simulink model "Simulation"  (R2019b)
settings: Solver=VariableStepAuto  StartTime=0.0  StopTime=150  RelTol=1e-3
values from neighbouring files (symbols this model uses):
  A = [1 1 1 1 ... (first row only)    [Parameters.m]
  actuator_calculator = [ ... (first row only)    [Parameters.m]
  cl = 0.0000002    (= 2e-07)    [Parameters.m]
  g = -9.81    [Parameters.m]
  ground_level = 0    [Parameters.m]
  Ixx = 0.2    [Parameters.m]
  Iyy = 0.2    [Parameters.m]
  Izz = 0.2    [Parameters.m]
  m = 2.2    [Parameters.m]
  maxLiftForce = maxRPM^2 * cl    (= 20)    [Parameters.m]
  P = [0 0 0 0 ... (first row only)    [Parameters.m]
  Pos_init = [0;0;0]    [Parameters.m]
  Vel_init = [0;0;0]    [Parameters.m]
libraries: simulink x12, sharedtransform x6, dspsolvers x2, sharedutil x1, aerolibutil x1, aerolibnav x1
settings Model: Creator=Szabolcs  LastModifiedBy=Szabolcs
settings SolverCC: ZeroCrossAlgorithm=Adaptive
settings DebuggingCC: IgnoredZcDiagnostic=none

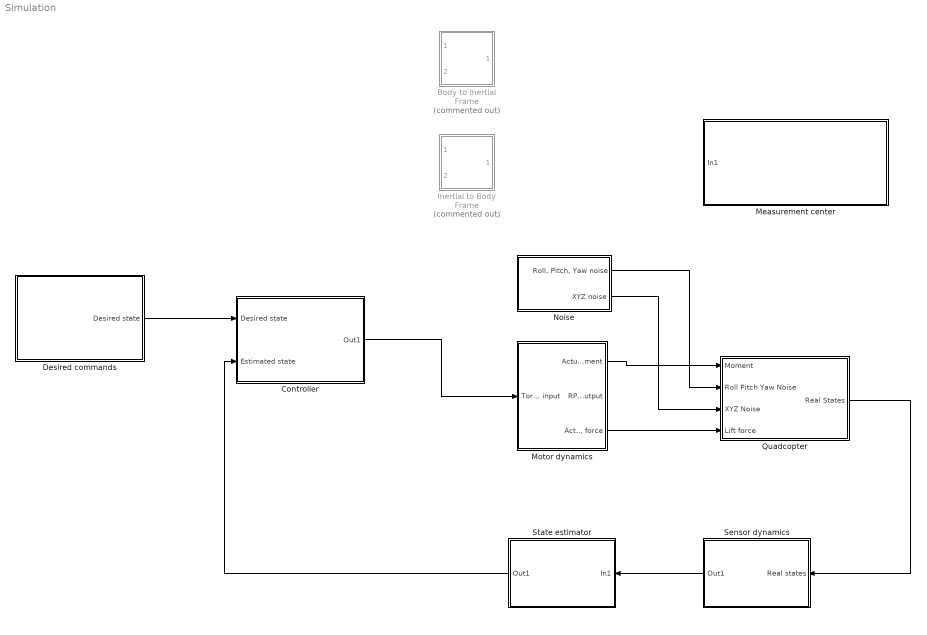
== system Simulation ==
  Body to Inertial Frame : Subsystem  Commented=on
  Controller : Subsystem
  Desired commands : Subsystem
  Inertial to Body Frame : Subsystem  Commented=on
  Measurement center : Subsystem
  Motor dynamics : Subsystem
  Noise : Subsystem
  Quadcopter : Subsystem
  Sensor dynamics : Subsystem
  State estimator : Subsystem
  wires:
  Quadcopter/1(Real States) -> Sensor dynamics/1(Real states)
  Sensor dynamics/1(Out1) -> State estimator/1(In1)
  Motor dynamics/3(Actuator Lift force) -> Quadcopter/4(Lift force)
  Motor dynamics/1(Actuator Moment) -> Quadcopter/1(Moment)
  Noise/2(XYZ noise) -> Quadcopter/3(XYZ Noise)
  Noise/1("Roll, Pitch, Yaw noise") -> Quadcopter/2(Roll Pitch Yaw Noise)
  Desired commands/1(Desired state) -> Controller/1(Desired state)
  State estimator/1(Out1) -> Controller/2(Estimated state)
  Controller/1(Out1) -> Motor dynamics/1(Torque input)

== system Simulation/Body to Inertial Frame ==
  Angles : Inport
  Inertial Vector : Inport  Port=2
  Matrix Multiply : Product  Multiplication=Matrix(*)
  Rotation Angles to Direction Cosine Matrix : sharedtransform/Rotation Angles to Direction Cosine Matrix  rotationOrder=ZYX  aMode=aMode
      settings: SourceProductBaseCode=AE
  Selector3 : Selector  InputPortWidth=3  IndexOptions=Index vector (dialog)  Indices=[3 2 1]  OutputSizes=1
  Transpose : Math  Operator=transpose  RndMeth=Zero  SaturateOnIntegerOverflow=on
  Body Vector : Outport
  wires:
  Rotation Angles to Direction Cosine Matrix/1 -> Transpose/1
  Selector3/1 -> Rotation Angles to Direction Cosine Matrix/1
  Angles/1 -> Selector3/1
  Matrix Multiply/1 -> Body Vector/1
  Inertial Vector/1 -> Matrix Multiply/2
  Transpose/1 -> Matrix Multiply/1

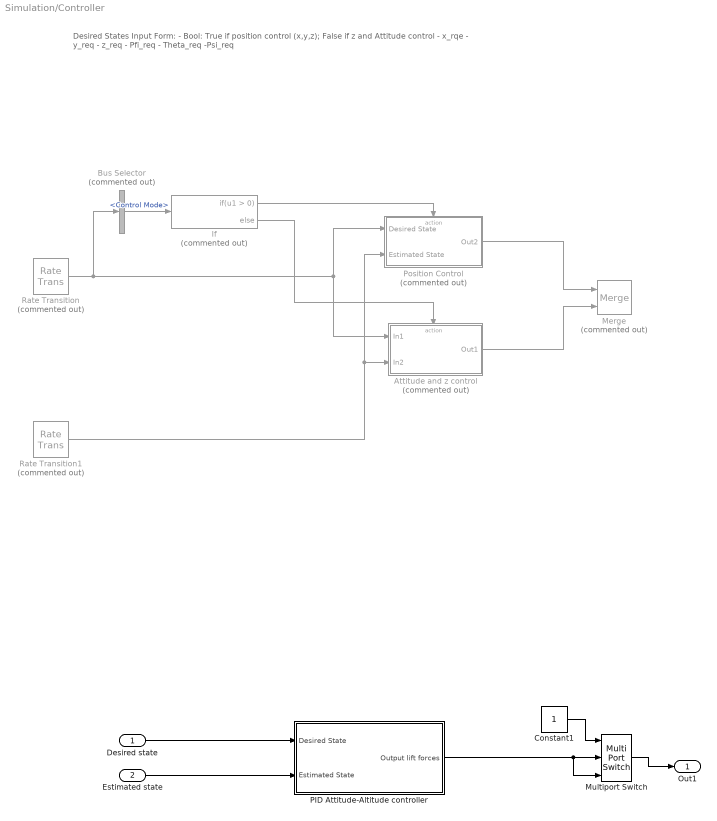
== system Simulation/Controller ==
  note: Desired States Input Form:
      | - Bool: True if position control (x,y,z); False if z and Attitude control
      | - x_rqe
      | - y_req
      | - z_req
      | - Pfi_req
      | - Theta_req
      | -Psi_req
  Desired state : Inport
  Estimated state : Inport  Port=2
  Attitude and z control : Subsystem  Commented=on  TreatAsAtomicUnit=on
  Bus Selector : BusSelector  Commented=on  OutputSignals=Control Mode
  Constant1 : Constant
  If : If  Commented=on
  Merge : Merge  Commented=on
  Multiport Switch : MultiPortSwitch  Inputs=2
  PID Attitude-Altitude controller : Subsystem
  Position Control : Subsystem  Commented=on  TreatAsAtomicUnit=on
  Rate Transition : RateTransition  Commented=on
  Rate Transition1 : RateTransition  Commented=on
  Out1 : Outport
  wires:
  Attitude and z control/1(Out1) -> Merge/2
  Position Control/1(Out2) -> Merge/1
  Bus Selector/1 -> If/1  "<Control Mode>"
  If/1 -> Position Control/Action
  If/2 -> Attitude and z control/Action
  Rate Transition/1 -> Position Control/1(Desired State), Attitude and z control/1(In1), Bus Selector/1
  Rate Transition1/1 -> Position Control/2(Estimated State), Attitude and z control/2(In2)
  Multiport Switch/1 -> Out1/1
  Constant1/1 -> Multiport Switch/1
  Desired state/1 -> PID Attitude-Altitude controller/1(Desired State)
  Estimated state/1 -> PID Attitude-Altitude controller/2(Estimated State)
  PID Attitude-Altitude controller/1(Output lift forces) -> Multiport Switch/3, Multiport Switch/2

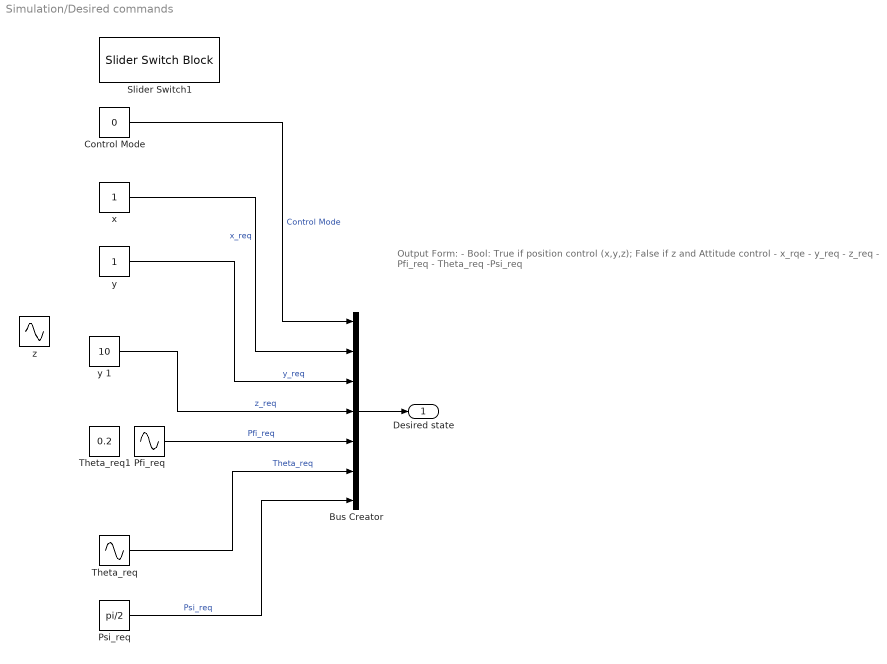
== system Simulation/Desired commands ==
  note: Output Form:
      | - Bool: True if position control (x,y,z); False if z and Attitude control
      | - x_rqe
      | - y_req
      | - z_req
      | - Pfi_req
      | - Theta_req
      | -Psi_req
  Bus Creator : BusCreator  Inputs=7
  Control Mode : Constant  Value=0
  Pfi_req : Sin  Amplitude=pi/6  Frequency=pi/10  SampleTime=0
  Psi_req : Constant  Value=pi/2
  Slider Switch1 : SliderSwitchBlock
      settings: Values={{'Off', 'On'}, [0 1]}
  Theta_req : Sin  Amplitude=pi/6  Frequency=pi/10  SampleTime=0
  Theta_req1 : Constant  Value=0.2
  x : Constant
  "y " : Constant
  y 1 : Constant  Value=10
  z : Sin  Amplitude=2  Bias=4  Frequency=pi/2  SampleTime=0
  Desired state : Outport
  wires:
  Psi_req/1 -> Bus Creator/7  "Psi_req"
  Bus Creator/1 -> Desired state/1
  Theta_req/1 -> Bus Creator/6  "Theta_req"
  "y "/1 -> Bus Creator/3  "y_req"
  Control Mode/1 -> Bus Creator/1  "Control Mode"
  x/1 -> Bus Creator/2  "x_req"
  y 1/1 -> Bus Creator/4  "z_req"
  Pfi_req/1 -> Bus Creator/5  "Pfi_req"

== system Simulation/Inertial to Body Frame ==
  Angles : Inport
  Inertial Vector : Inport  Port=2
  Matrix Multiply : Product  Multiplication=Matrix(*)
  Rotation Angles to Direction Cosine Matrix : sharedtransform/Rotation Angles to Direction Cosine Matrix  rotationOrder=ZYX  aMode=aMode
      settings: SourceProductBaseCode=AE
  Selector3 : Selector  InputPortWidth=3  IndexOptions=Index vector (dialog)  Indices=[3 2 1]  OutputSizes=1
  Body Vector : Outport
  wires:
  Selector3/1 -> Rotation Angles to Direction Cosine Matrix/1
  Angles/1 -> Selector3/1
  Matrix Multiply/1 -> Body Vector/1
  Inertial Vector/1 -> Matrix Multiply/2
  Rotation Angles to Direction Cosine Matrix/1 -> Matrix Multiply/1

== system Simulation/Measurement center ==
  In1 : Inport

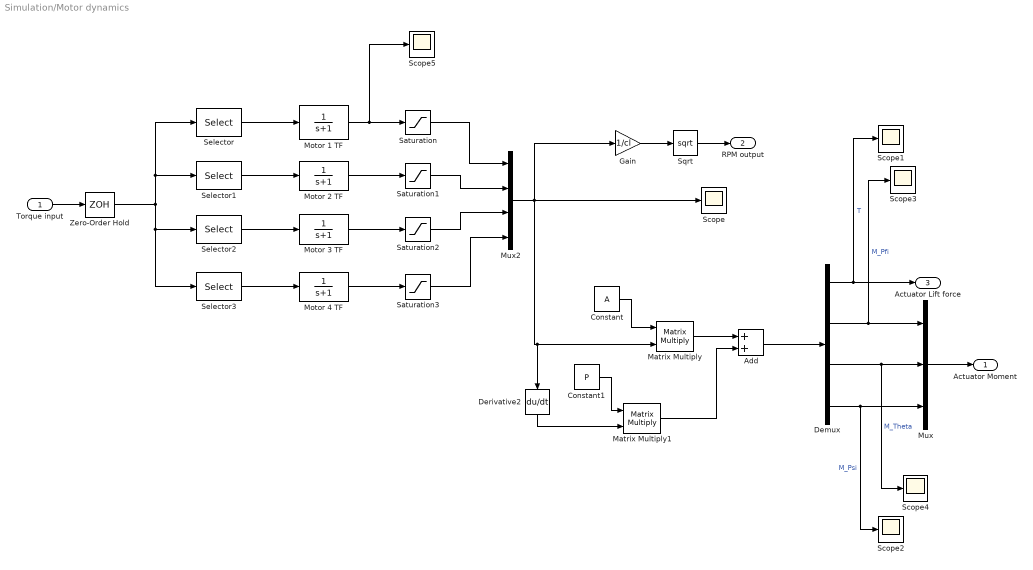
== system Simulation/Motor dynamics ==
  Torque input : Inport
  Add : Sum
  Constant : Constant  Value=A
  Constant1 : Constant  Value=P
  Demux : Demux
  Derivative2 : Derivative
  Gain : Gain  Gain=1/cl
  Matrix Multiply : Product  Multiplication=Matrix(*)
  Matrix Multiply1 : Product  Multiplication=Matrix(*)
  Motor 1 TF : TransferFcn  Denominator=[1 1]
  Motor 2 TF : TransferFcn  Denominator=[1 1]
  Motor 3 TF : TransferFcn  Denominator=[1 1]
  Motor 4 TF : TransferFcn  Denominator=[1 1]
  Mux : Mux  Inputs=3
  Mux2 : Mux
  Saturation{,1..3} (4 alike) : Saturate  UpperLimit=20  LowerLimit=0
  Scope{,1..5} (6 alike) : Scope
  Selector : Selector  InputPortWidth=4  IndexOptions=Index vector (dialog)  Indices=1  OutputSizes=1
  Selector1 : Selector  InputPortWidth=4  IndexOptions=Index vector (dialog)  Indices=2  OutputSizes=1
  Selector2 : Selector  InputPortWidth=4  IndexOptions=Index vector (dialog)  Indices=3  OutputSizes=1
  Selector3 : Selector  InputPortWidth=4  IndexOptions=Index vector (dialog)  Indices=4  OutputSizes=1
  Sqrt : Sqrt  SaturateOnIntegerOverflow=on
  Zero-Order Hold : ZeroOrderHold  SampleTime=0.01
  Actuator Moment : Outport
  RPM output : Outport  Port=2
  Actuator Lift force : Outport  Port=3
  wires:
  Selector/1 -> Motor 1 TF/1
  Selector1/1 -> Motor 2 TF/1
  Zero-Order Hold/1 -> Selector3/1, Selector2/1, Selector1/1, Selector/1
  Torque input/1 -> Zero-Order Hold/1
  Saturation/1 -> Mux2/1
  Saturation1/1 -> Mux2/2
  Selector3/1 -> Motor 4 TF/1
  Saturation3/1 -> Mux2/4
  Saturation2/1 -> Mux2/3
  Motor 1 TF/1 -> Scope5/1, Saturation/1
  Motor 3 TF/1 -> Saturation2/1
  Motor 4 TF/1 -> Saturation3/1
  Motor 2 TF/1 -> Saturation1/1
  Selector2/1 -> Motor 3 TF/1
  Mux2/1 -> Gain/1, Derivative2/1, Matrix Multiply/2, Scope/1
  Constant/1 -> Matrix Multiply/1
  Constant1/1 -> Matrix Multiply1/1
  Derivative2/1 -> Matrix Multiply1/2
  Mux/1 -> Actuator Moment/1
  Sqrt/1 -> RPM output/1
  Gain/1 -> Sqrt/1
  Matrix Multiply1/1 -> Add/2
  Demux/1 -> Scope1/1, Actuator Lift force/1  "T"
  Demux/4 -> Scope2/1, Mux/3  "M_Psi"
  Demux/2 -> Scope3/1, Mux/1  "M_Pfi"
  Demux/3 -> Mux/2, Scope4/1  "M_Theta"
  Matrix Multiply/1 -> Add/1
  Add/1 -> Demux/1

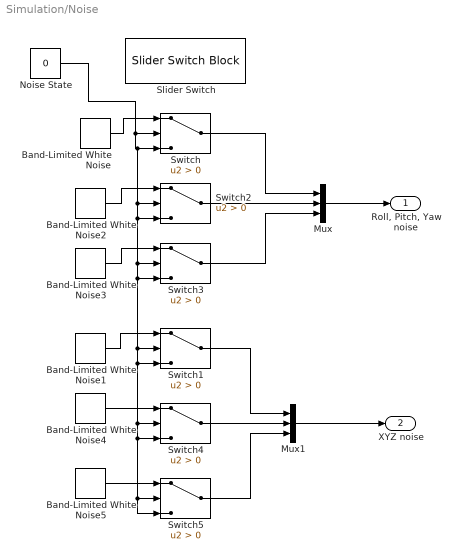
== system Simulation/Noise ==
  Band-Limited White Noise{,1..5} (6 alike) : simulink/Sources/Band-Limited White Noise  Cov=[1]  Ts=0.1  seed=[23341]
  Mux : Mux  Inputs=3
  Mux1 : Mux  Inputs=3
  Noise State : Constant  Value=0
  Slider Switch : SliderSwitchBlock
      settings: Values={{'Off', 'On'}, [0 1]}
  Switch{,1..5} (6 alike) : Switch  Criteria=u2 > Threshold
  "Roll, Pitch, Yaw noise" : Outport
  XYZ noise : Outport  Port=2
  wires:
  Noise State/1 -> Switch2/2, Switch2/3, Switch3/2, Switch3/3, Switch5/3, Switch5/2, Switch4/3, Switch4/2, Switch1/3, Switch1/2, Switch/3, Switch/2
  Band-Limited White Noise/1 -> Switch/1
  Band-Limited White Noise1/1 -> Switch1/1
  Mux/1 -> "Roll, Pitch, Yaw noise"/1
  Switch/1 -> Mux/1
  Switch2/1 -> Mux/2
  Switch3/1 -> Mux/3
  Band-Limited White Noise3/1 -> Switch3/1
  Band-Limited White Noise2/1 -> Switch2/1
  Switch4/1 -> Mux1/2
  Switch1/1 -> Mux1/1
  Switch5/1 -> Mux1/3
  Mux1/1 -> XYZ noise/1
  Band-Limited White Noise4/1 -> Switch4/1
  Band-Limited White Noise5/1 -> Switch5/1

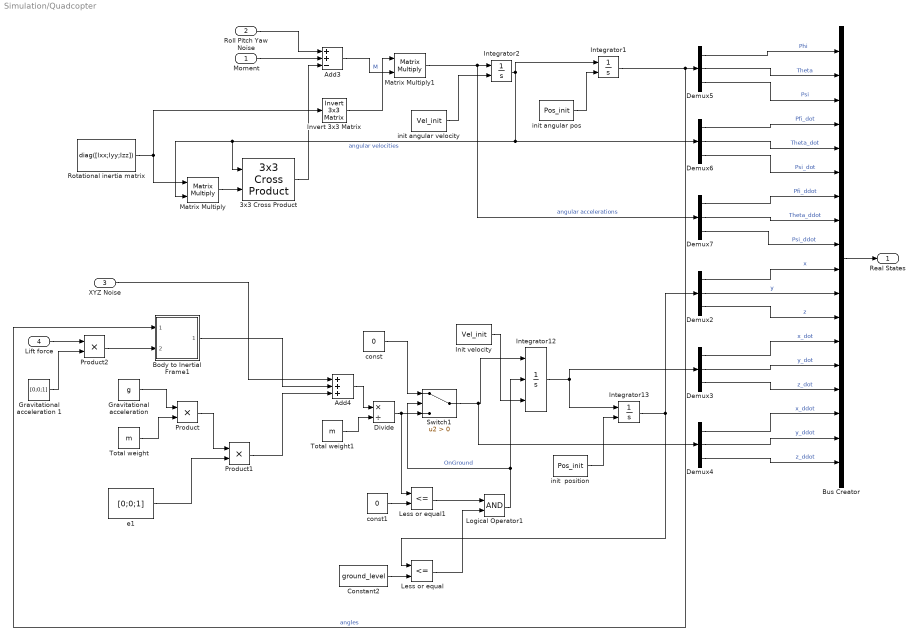
== system Simulation/Quadcopter ==
  Moment : Inport
  Roll Pitch Yaw Noise : Inport  Port=2
  XYZ Noise : Inport  Port=3
  Lift force : Inport  Port=4
  3x3 Cross Product : sharedutil/3x3 Cross Product  aMode=aMode
      settings: SourceProductBaseCode=AE
  Add3 : Sum  Inputs=++-
  Add4 : Sum  Inputs=+++
  Body to Inertial Frame1 : Subsystem
  Bus Creator : BusCreator  Inputs=18
  Constant2 : Constant  Value=ground_level
  Demux{2..7} (6 alike) : Demux  Outputs=3
  Divide : Product  Inputs=*/
  "Gravitational acceleration " : Constant  Value=g
  Gravitational acceleration 1 : Constant  Value=[0;0;1]
  Init velocity : Constant  Value=Vel_init
  Integrator1 : Integrator  InitialConditionSource=external
  Integrator12 : Integrator  ExternalReset=rising  InitialConditionSource=external
  Integrator13 : Integrator  InitialConditionSource=external
  Integrator2 : Integrator  InitialConditionSource=external
  Invert 3x3 Matrix : aerolibutil/Invert  3x3 Matrix
  Less or equal : RelationalOperator  Operator=<=  OutDataTypeStr=boolean  RndMeth=Simplest
  Less or equal1 : RelationalOperator  Operator=<=  OutDataTypeStr=boolean  RndMeth=Simplest
  Logical Operator1 : Logic  AllPortsSameDT=off  OutDataTypeStr=boolean
  Matrix Multiply : Product  Multiplication=Matrix(*)
  Matrix Multiply1 : Product  Multiplication=Matrix(*)
  Product : Product
  Product1 : Product
  Product2 : Product
  Rotational inertia matrix : Constant  Value=diag([Ixx;Iyy;Izz])
  Switch1 : Switch  Criteria=u2 > Threshold
  Total weight : Constant  Value=m
  Total weight1 : Constant  Value=m
  const : Constant  Value=0
  const1 : Constant  Value=0
  e1 : Constant  Value=[0;0;1]
  init  position : Constant  Value=Pos_init
  init angular pos : Constant  Value=Pos_init
  init angular velocity : Constant  Value=Vel_init
  Real States : Outport
  wires:
  Constant2/1 -> Less or equal/2
  Total weight1/1 -> Divide/2
  Integrator13/1 -> Less or equal/1, Demux2/1
  Divide/1 -> Less or equal1/1, Switch1/3
  const1/1 -> Less or equal1/2
  Product1/1 -> Add4/3
  e1/1 -> Product1/2
  Product/1 -> Product1/1
  Switch1/1 -> Demux4/1, Integrator12/1
  Logical Operator1/1 -> Switch1/2, Integrator12/2  "OnGround"
  Total weight/1 -> Product/2
  const/1 -> Switch1/1
  Body to Inertial Frame1/1(Body Vector) -> Add4/2
  Less or equal1/1 -> Logical Operator1/1
  "Gravitational acceleration "/1 -> Product/1
  Less or equal/1 -> Logical Operator1/2
  Add4/1 -> Divide/1
  XYZ Noise/1 -> Add4/1
  Integrator2/1 -> Integrator1/1, Demux6/1, 3x3 Cross Product/1, Matrix Multiply/2  "angular velocities"
  Integrator1/1 -> Body to Inertial Frame1/1(Angles), Demux5/1  "angles"
  Rotational inertia matrix/1 -> Matrix Multiply/1, Invert 3x3 Matrix/1
  Matrix Multiply1/1 -> Integrator2/1, Demux7/1  "angular accelerations"
  Roll Pitch Yaw Noise/1 -> Add3/1
  Moment/1 -> Add3/2
  Add3/1 -> Matrix Multiply1/2  "M"
  Invert 3x3 Matrix/1 -> Matrix Multiply1/1
  3x3 Cross Product/1 -> Add3/3
  Matrix Multiply/1 -> 3x3 Cross Product/2
  init angular velocity/1 -> Integrator2/2
  init angular pos/1 -> Integrator1/2
  Init velocity/1 -> Integrator12/3
  init  position/1 -> Integrator13/2
  Integrator12/1 -> Integrator13/1, Demux3/1
  Bus Creator/1 -> Real States/1
  Demux5/1 -> Bus Creator/1  "Phi"
  Demux5/2 -> Bus Creator/2  "Theta"
  Demux5/3 -> Bus Creator/3  "Psi"
  Demux6/1 -> Bus Creator/4  "Pfi_dot"
  Demux6/2 -> Bus Creator/5  "Theta_dot"
  Demux6/3 -> Bus Creator/6  "Psi_dot"
  Demux7/1 -> Bus Creator/7  "Pfi_ddot"
  Demux7/2 -> Bus Creator/8  "Theta_ddot"
  Demux7/3 -> Bus Creator/9  "Psi_ddot"
  Demux2/1 -> Bus Creator/10  "x"
  Demux2/2 -> Bus Creator/11  "y"
  Demux2/3 -> Bus Creator/12  "z"
  Demux3/1 -> Bus Creator/13  "x_dot"
  Demux3/2 -> Bus Creator/14  "y_dot"
  Demux3/3 -> Bus Creator/15  "z_dot"
  Demux4/1 -> Bus Creator/16  "x_ddot"
  Demux4/2 -> Bus Creator/17  "y_ddot"
  Demux4/3 -> Bus Creator/18  "z_ddot"
  Lift force/1 -> Product2/1
  Product2/1 -> Body to Inertial Frame1/2(Inertial Vector)
  Gravitational acceleration 1/1 -> Product2/2

== system Simulation/Sensor dynamics ==
  Real states : Inport
  Advanced sensor behavious simulation : Constant  Value=0
  Detailed sensor behaviour : Subsystem
  Simplified sensor behaviour : Subsystem
  Slider Switch : SliderSwitchBlock
      settings: Values={{'Off', 'On'}, [0 1]}
  Switch1 : Switch  Criteria=u2 > Threshold
  Out1 : Outport
  wires:
  Switch1/1 -> Out1/1
  Advanced sensor behavious simulation/1 -> Switch1/2
  Real states/1 -> Simplified sensor behaviour/1(Real states), Detailed sensor behaviour/1(In1)
  Simplified sensor behaviour/1(Sensor output) -> Switch1/1, Switch1/3

== system Simulation/State estimator ==
  In1 : Inport
  Ideal State estimator : Subsystem
  Ideal state estimator / Kalman filter : Constant  Value=0
  Slider Switch : SliderSwitchBlock
      settings: Values={{'Off', 'On'}, [0 1]}
  Switch1 : Switch  Criteria=u2 > Threshold
  Out1 : Outport
  wires:
  Switch1/1 -> Out1/1
  In1/1 -> Ideal State estimator/1(In1)
  Ideal State estimator/1(Out1) -> Switch1/3, Switch1/1
  Ideal state estimator / Kalman filter/1 -> Switch1/2

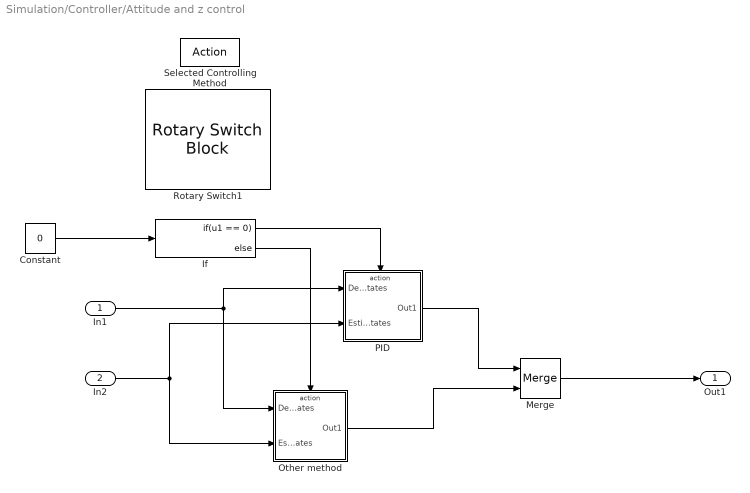
== system Simulation/Controller/Attitude and z control ==
  In1 : Inport
  In2 : Inport  Port=2
  Selected Controlling Method : ActionPort  ActionPortLabel=else
  Constant : Constant  Value=0
  If : If  IfExpression=u1 == 0
  Merge : Merge
  Other method : Subsystem  TreatAsAtomicUnit=on
  PID : Subsystem  TreatAsAtomicUnit=on
  Rotary Switch1 : RotarySwitchBlock
      settings: Values={{'PID', 'Low', 'Medium', 'High'}, [0 1 2 3]}
  Out1 : Outport
  wires:
  If/2 -> Other method/Action
  Merge/1 -> Out1/1
  PID/1(Out1) -> Merge/1
  In1/1 -> Other method/1(Desired States), PID/1(Desired States)
  In2/1 -> PID/2(Estimated States), Other method/2(Estimated States)
  Other method/1(Out1) -> Merge/2
  If/1 -> PID/Action
  Constant/1 -> If/1

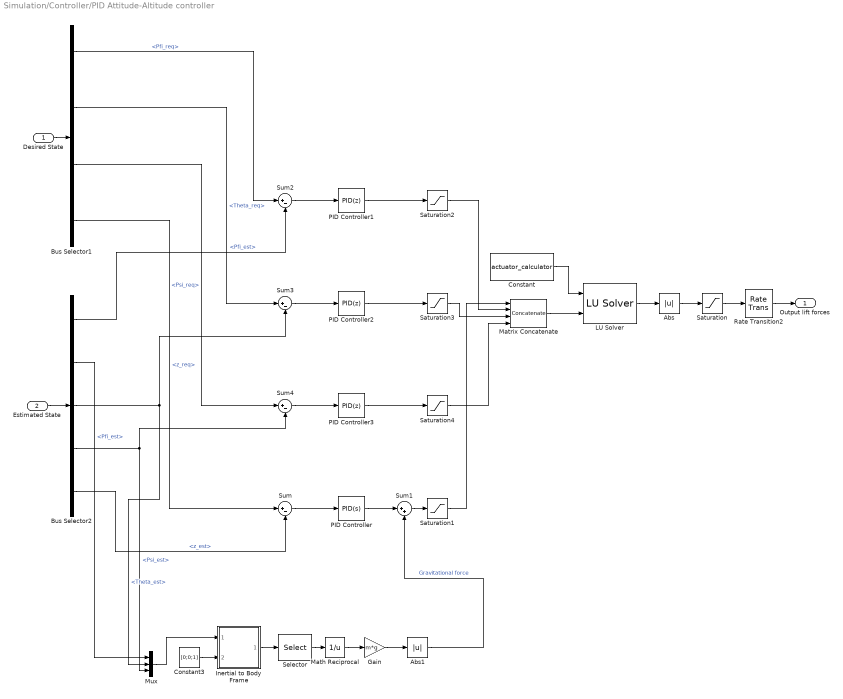
== system Simulation/Controller/PID Attitude-Altitude controller ==
  Desired State : Inport
  Estimated State : Inport  Port=2
  Abs : Abs
  Abs1 : Abs
  Bus Selector1 : BusSelector  OutputSignals=Pfi_req,Theta_req,Psi_req,z_req
  Bus Selector2 : BusSelector  OutputSignals=Pfi_est,Pfi_est,Theta_est,Psi_est,z_est
  Constant : Constant  Value=actuator_calculator
  Constant3 : Constant  Value=[0;0;1]
  Gain : Gain  Gain=m*g
  Inertial to Body Frame : Subsystem
  LU Solver : dspsolvers/LU Solver
      settings: SourceProductName=DSP System Toolbox  SourceProductBaseCode=DS
  Math Reciprocal : Math  Operator=reciprocal  SaturateOnIntegerOverflow=on
  Matrix Concatenate : Concatenate  NumInputs=4
  Mux : Mux  Inputs=3
  PID Controller : simulink/Continuous/PID Controller  Controller=PID  Form=Parallel  TimeDomain=Continuous-time  SampleTime=0.01  IntegratorMethod=Forward Euler  FilterMethod=Forward Euler  ControllerParametersSource=internal  P=0.22  I=0.000000001  D=1  UseFilter=on  N=100  TunerSelectOption=Transfer Function Based (PID Tuner App)  InitialConditionSource=internal  InitialConditionForIntegrator=0  InitialConditionForFilter=0  DifferentiatorICPrevScaledInput=0  ExternalReset=none  TrackingMode=off  Kt=1  LimitOutput=off  UpperSaturationLimit=inf  LowerSaturationLimit=-inf  LinearizeAsGain=on  AntiWindupMode=none  Kb=1  POutMin=[]  POutMax=[]  IOutMin=[]  IOutMax=[]  DOutMin=[]  DOutMax=[]  NOutMin=[]  NOutMax=[]  SumOutMin=[]  SumOutMax=[]  SaturationOutMin=[]  SaturationOutMax=[]  PParamMin=[]  PParamMax=[]  IParamMin=[]  IParamMax=[]  DParamMin=[]  DParamMax=[]  NParamMin=[]  NParamMax=[]  KbParamMin=[]  KbParamMax=[]  KtParamMin=[]  KtParamMax=[]  KbOutMin=[]  KbOutMax=[]  KtOutMin=[]  KtOutMax=[]  IntegratorOutMin=[]  IntegratorOutMax=[]  FilterOutMin=[]  FilterOutMax=[]  SumI1OutMin=[]  SumI1OutMax=[]  SumI2OutMin=[]  SumI2OutMax=[]  SumI3OutMin=[]  SumI3OutMax=[]  SumI4OutMin=[]  SumI4OutMax=[]  SumDOutMin=[]  SumDOutMax=[]  DifferentiatorOutMin=[]  DifferentiatorOutMax=[]  FilterDiffOutCoefMin=[]  FilterDiffOutCoefMax=[]  ReciprocalOutMin=[]  ReciprocalOutMax=[]  SumDenOutMin=[]  SumDenOutMax=[]  SumNumOutMin=[]  SumNumOutMax=[]  DivideOutMin=[]  DivideOutMax=[]  IntegratorContinuousStateAttributes=''  IntegratorStateMustResolveToSignalObject=off  IntegratorRTWStateStorageClass=Auto  FilterContinuousStateAttributes=''  FilterStateMustResolveToSignalObject=off  FilterRTWStateStorageClass=Auto  ParallelPVariant=InternalParameters  IdealPVariant=Disabled  IVariant=InternalParameters  DVariant=InternalParameters  IntegratorVariant=Continuous  SatVariant=Disabled  AWVariant=Passthrough  PCopyVariant=Disabled  TRVariant=Disabled  FdbkBlocksVariant=Forward  IdealPFdbkVariant=Disabled  SatFdbkVariant=Disabled  DerivativeFilterVariant=ContFilter  NVariant=InternalParameters  NCopyVariant=Disabled  FilterICVariant=InternalICsFilter  IntegratorICVariant=InternalICs  ExternalResetVariant=Disabled  TRSumVariant=Passthrough  SumFdbkVariant=Disabled  SumVariant=Sum_PID
  PID Controller1 : simulink/Continuous/PID Controller  Controller=PID  Form=Parallel  TimeDomain=Discrete-time  SampleTime=0.01  IntegratorMethod=Forward Euler  FilterMethod=Forward Euler  ControllerParametersSource=internal  P=0.00204890385196012  I=6.86634656190928e-06  D=0.114572255070436  UseFilter=on  N=45.1692938598137  TunerSelectOption=Transfer Function Based (PID Tuner App)  InitialConditionSource=internal  InitialConditionForIntegrator=0  InitialConditionForFilter=0  DifferentiatorICPrevScaledInput=0  ExternalReset=none  TrackingMode=off  Kt=1  LimitOutput=off  UpperSaturationLimit=inf  LowerSaturationLimit=-inf  LinearizeAsGain=on  AntiWindupMode=none  Kb=1  POutMin=[]  POutMax=[]  IOutMin=[]  IOutMax=[]  DOutMin=[]  DOutMax=[]  NOutMin=[]  NOutMax=[]  SumOutMin=[]  SumOutMax=[]  SaturationOutMin=[]  SaturationOutMax=[]  PParamMin=[]  PParamMax=[]  IParamMin=[]  IParamMax=[]  DParamMin=[]  DParamMax=[]  NParamMin=[]  NParamMax=[]  KbParamMin=[]  KbParamMax=[]  KtParamMin=[]  KtParamMax=[]  KbOutMin=[]  KbOutMax=[]  KtOutMin=[]  KtOutMax=[]  IntegratorOutMin=[]  IntegratorOutMax=[]  FilterOutMin=[]  FilterOutMax=[]  SumI1OutMin=[]  SumI1OutMax=[]  SumI2OutMin=[]  SumI2OutMax=[]  SumI3OutMin=[]  SumI3OutMax=[]  SumI4OutMin=[]  SumI4OutMax=[]  SumDOutMin=[]  SumDOutMax=[]  DifferentiatorOutMin=[]  DifferentiatorOutMax=[]  FilterDiffOutCoefMin=[]  FilterDiffOutCoefMax=[]  ReciprocalOutMin=[]  ReciprocalOutMax=[]  SumDenOutMin=[]  SumDenOutMax=[]  SumNumOutMin=[]  SumNumOutMax=[]  DivideOutMin=[]  DivideOutMax=[]  IntegratorContinuousStateAttributes=''  IntegratorStateMustResolveToSignalObject=off  IntegratorRTWStateStorageClass=Auto  FilterContinuousStateAttributes=''  FilterStateMustResolveToSignalObject=off  FilterRTWStateStorageClass=Auto  ParallelPVariant=InternalParameters  IdealPVariant=Disabled  IVariant=InternalParameters  DVariant=InternalParameters  IntegratorVariant=Discrete  SatVariant=Disabled  AWVariant=Passthrough  PCopyVariant=Disabled  TRVariant=Disabled  FdbkBlocksVariant=Forward  IdealPFdbkVariant=Disabled  SatFdbkVariant=Disabled  DerivativeFilterVariant=ForwardEulerFilter  NVariant=InternalParameters  NCopyVariant=Disabled  FilterICVariant=InternalICsFilter  IntegratorICVariant=InternalICs  ExternalResetVariant=Disabled  TRSumVariant=Passthrough  SumFdbkVariant=Disabled  SumVariant=Sum_PID
  PID Controller2 : simulink/Continuous/PID Controller  Controller=PID  Form=Parallel  TimeDomain=Discrete-time  SampleTime=0.01  IntegratorMethod=Forward Euler  FilterMethod=Forward Euler  ControllerParametersSource=internal  P=0.0140402401976709  I=0.000105041222491544  D=0.416944052852644  UseFilter=on  N=84.580517531451  TunerSelectOption=Transfer Function Based (PID Tuner App)  InitialConditionSource=internal  InitialConditionForIntegrator=0  InitialConditionForFilter=0  DifferentiatorICPrevScaledInput=0  ExternalReset=none  TrackingMode=off  Kt=1  LimitOutput=off  UpperSaturationLimit=inf  LowerSaturationLimit=-inf  LinearizeAsGain=on  AntiWindupMode=none  Kb=1  POutMin=[]  POutMax=[]  IOutMin=[]  IOutMax=[]  DOutMin=[]  DOutMax=[]  NOutMin=[]  NOutMax=[]  SumOutMin=[]  SumOutMax=[]  SaturationOutMin=[]  SaturationOutMax=[]  PParamMin=[]  PParamMax=[]  IParamMin=[]  IParamMax=[]  DParamMin=[]  DParamMax=[]  NParamMin=[]  NParamMax=[]  KbParamMin=[]  KbParamMax=[]  KtParamMin=[]  KtParamMax=[]  KbOutMin=[]  KbOutMax=[]  KtOutMin=[]  KtOutMax=[]  IntegratorOutMin=[]  IntegratorOutMax=[]  FilterOutMin=[]  FilterOutMax=[]  SumI1OutMin=[]  SumI1OutMax=[]  SumI2OutMin=[]  SumI2OutMax=[]  SumI3OutMin=[]  SumI3OutMax=[]  SumI4OutMin=[]  SumI4OutMax=[]  SumDOutMin=[]  SumDOutMax=[]  DifferentiatorOutMin=[]  DifferentiatorOutMax=[]  FilterDiffOutCoefMin=[]  FilterDiffOutCoefMax=[]  ReciprocalOutMin=[]  ReciprocalOutMax=[]  SumDenOutMin=[]  SumDenOutMax=[]  SumNumOutMin=[]  SumNumOutMax=[]  DivideOutMin=[]  DivideOutMax=[]  IntegratorContinuousStateAttributes=''  IntegratorStateMustResolveToSignalObject=off  IntegratorRTWStateStorageClass=Auto  FilterContinuousStateAttributes=''  FilterStateMustResolveToSignalObject=off  FilterRTWStateStorageClass=Auto  ParallelPVariant=InternalParameters  IdealPVariant=Disabled  IVariant=InternalParameters  DVariant=InternalParameters  IntegratorVariant=Discrete  SatVariant=Disabled  AWVariant=Passthrough  PCopyVariant=Disabled  TRVariant=Disabled  FdbkBlocksVariant=Forward  IdealPFdbkVariant=Disabled  SatFdbkVariant=Disabled  DerivativeFilterVariant=ForwardEulerFilter  NVariant=InternalParameters  NCopyVariant=Disabled  FilterICVariant=InternalICsFilter  IntegratorICVariant=InternalICs  ExternalResetVariant=Disabled  TRSumVariant=Passthrough  SumFdbkVariant=Disabled  SumVariant=Sum_PID
  PID Controller3 : simulink/Continuous/PID Controller  Controller=PID  Form=Parallel  TimeDomain=Discrete-time  SampleTime=0.01  IntegratorMethod=Forward Euler  FilterMethod=Forward Euler  ControllerParametersSource=internal  P=0.0478772088635547  I=0.000562502871315751  D=0.905321531273544  UseFilter=on  N=107.012641004188  TunerSelectOption=Transfer Function Based (PID Tuner App)  InitialConditionSource=internal  InitialConditionForIntegrator=0  InitialConditionForFilter=0  DifferentiatorICPrevScaledInput=0  ExternalReset=none  TrackingMode=off  Kt=1  LimitOutput=off  UpperSaturationLimit=inf  LowerSaturationLimit=-inf  LinearizeAsGain=on  AntiWindupMode=none  Kb=1  POutMin=[]  POutMax=[]  IOutMin=[]  IOutMax=[]  DOutMin=[]  DOutMax=[]  NOutMin=[]  NOutMax=[]  SumOutMin=[]  SumOutMax=[]  SaturationOutMin=[]  SaturationOutMax=[]  PParamMin=[]  PParamMax=[]  IParamMin=[]  IParamMax=[]  DParamMin=[]  DParamMax=[]  NParamMin=[]  NParamMax=[]  KbParamMin=[]  KbParamMax=[]  KtParamMin=[]  KtParamMax=[]  KbOutMin=[]  KbOutMax=[]  KtOutMin=[]  KtOutMax=[]  IntegratorOutMin=[]  IntegratorOutMax=[]  FilterOutMin=[]  FilterOutMax=[]  SumI1OutMin=[]  SumI1OutMax=[]  SumI2OutMin=[]  SumI2OutMax=[]  SumI3OutMin=[]  SumI3OutMax=[]  SumI4OutMin=[]  SumI4OutMax=[]  SumDOutMin=[]  SumDOutMax=[]  DifferentiatorOutMin=[]  DifferentiatorOutMax=[]  FilterDiffOutCoefMin=[]  FilterDiffOutCoefMax=[]  ReciprocalOutMin=[]  ReciprocalOutMax=[]  SumDenOutMin=[]  SumDenOutMax=[]  SumNumOutMin=[]  SumNumOutMax=[]  DivideOutMin=[]  DivideOutMax=[]  IntegratorContinuousStateAttributes=''  IntegratorStateMustResolveToSignalObject=off  IntegratorRTWStateStorageClass=Auto  FilterContinuousStateAttributes=''  FilterStateMustResolveToSignalObject=off  FilterRTWStateStorageClass=Auto  ParallelPVariant=InternalParameters  IdealPVariant=Disabled  IVariant=InternalParameters  DVariant=InternalParameters  IntegratorVariant=Discrete  SatVariant=Disabled  AWVariant=Passthrough  PCopyVariant=Disabled  TRVariant=Disabled  FdbkBlocksVariant=Forward  IdealPFdbkVariant=Disabled  SatFdbkVariant=Disabled  DerivativeFilterVariant=ForwardEulerFilter  NVariant=InternalParameters  NCopyVariant=Disabled  FilterICVariant=InternalICsFilter  IntegratorICVariant=InternalICs  ExternalResetVariant=Disabled  TRSumVariant=Passthrough  SumFdbkVariant=Disabled  SumVariant=Sum_PID
  Rate Transition2 : RateTransition
  Saturation : Saturate  UpperLimit=maxLiftForce  LowerLimit=0
  Saturation1 : Saturate  UpperLimit=4 * maxLiftForce  LowerLimit=0
  Saturation2 : Saturate  UpperLimit=0.01  LowerLimit=-0.01
  Saturation3 : Saturate  UpperLimit=0.01  LowerLimit=-0.01
  Saturation4 : Saturate  UpperLimit=10  LowerLimit=-10
  Selector : Selector  InputPortWidth=3  IndexOptions=Index vector (dialog)  Indices=3  OutputSizes=1
  Sum{,2..4} (4 alike) : Sum  Inputs=|+-
  Sum1 : Sum  Inputs=|++
  Output lift forces : Outport
  wires:
  Gain/1 -> Abs1/1
  Saturation2/1 -> Matrix Concatenate/2
  Sum3/1 -> PID Controller2/1
  Bus Selector1/2 -> Sum3/1  "<Theta_req>"
  Selector/1 -> Math Reciprocal/1
  Sum4/1 -> PID Controller3/1
  Saturation/1 -> Rate Transition2/1
  PID Controller1/1 -> Saturation2/1
  Bus Selector1/3 -> Sum4/1  "<Psi_req>"
  Saturation3/1 -> Matrix Concatenate/3
  PID Controller3/1 -> Saturation4/1
  Bus Selector2/1 -> Sum2/2  "<Pfi_est>"
  Sum/1 -> PID Controller/1
  Desired State/1 -> Bus Selector1/1
  LU Solver/1 -> Abs/1
  PID Controller/1 -> Sum1/1
  Constant/1 -> LU Solver/1
  Saturation1/1 -> Matrix Concatenate/1
  PID Controller2/1 -> Saturation3/1
  Math Reciprocal/1 -> Gain/1
  Estimated State/1 -> Bus Selector2/1
  Abs1/1 -> Sum1/2  "Gravitational force"
  Inertial to Body Frame/1(Body Vector) -> Selector/1
  Bus Selector1/4 -> Sum/1  "<z_req>"
  Sum1/1 -> Saturation1/1
  Bus Selector2/2 -> Mux/1  "<Pfi_est>"
  Bus Selector1/1 -> Sum2/1  "<Pfi_req>"
  Bus Selector2/3 -> Mux/2, Sum3/2  "<Theta_est>"
  Bus Selector2/4 -> Mux/3, Sum4/2  "<Psi_est>"
  Saturation4/1 -> Matrix Concatenate/4
  Mux/1 -> Inertial to Body Frame/1(Angles)
  Constant3/1 -> Inertial to Body Frame/2(Inertial Vector)
  Sum2/1 -> PID Controller1/1
  Rate Transition2/1 -> Output lift forces/1
  Bus Selector2/5 -> Sum/2  "<z_est>"
  Matrix Concatenate/1 -> LU Solver/2
  Abs/1 -> Saturation/1

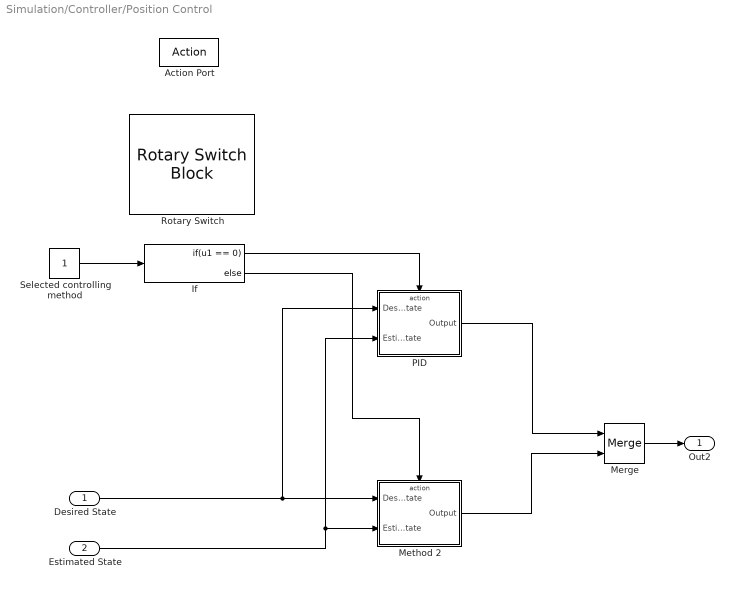
== system Simulation/Controller/Position Control ==
  Desired State : Inport
  Estimated State : Inport  Port=2
  Action Port : ActionPort  ActionPortLabel=if(u1 > 0)
  If : If  IfExpression=u1 == 0
  Merge : Merge
  Method 2 : Subsystem  TreatAsAtomicUnit=on
  PID : Subsystem  TreatAsAtomicUnit=on
  Rotary Switch : RotarySwitchBlock
      settings: Values={{'PID', 'Low', 'Medium', 'High'}, [0 1 2 3]}
  Selected controlling method : Constant
  Out2 : Outport
  wires:
  Selected controlling method/1 -> If/1
  Desired State/1 -> PID/1(Desired State), Method 2/1(Desired State)
  If/1 -> PID/Action
  Estimated State/1 -> PID/2(Estimated State), Method 2/2(Estimated State)
  Merge/1 -> Out2/1
  PID/1(Output) -> Merge/1
  Method 2/1(Output) -> Merge/2
  If/2 -> Method 2/Action

== system Simulation/Quadcopter/Body to Inertial Frame1 ==
  Angles : Inport
  Inertial Vector : Inport  Port=2
  Matrix Multiply : Product  Multiplication=Matrix(*)
  Rotation Angles to Direction Cosine Matrix : sharedtransform/Rotation Angles to Direction Cosine Matrix  rotationOrder=ZYX  aMode=aMode
      settings: SourceProductBaseCode=AE
  Selector3 : Selector  InputPortWidth=3  IndexOptions=Index vector (dialog)  Indices=[3 2 1]  OutputSizes=1
  Transpose : Math  Operator=transpose  RndMeth=Zero  SaturateOnIntegerOverflow=on
  Body Vector : Outport
  wires:
  Rotation Angles to Direction Cosine Matrix/1 -> Transpose/1
  Selector3/1 -> Rotation Angles to Direction Cosine Matrix/1
  Angles/1 -> Selector3/1
  Matrix Multiply/1 -> Body Vector/1
  Inertial Vector/1 -> Matrix Multiply/2
  Transpose/1 -> Matrix Multiply/1

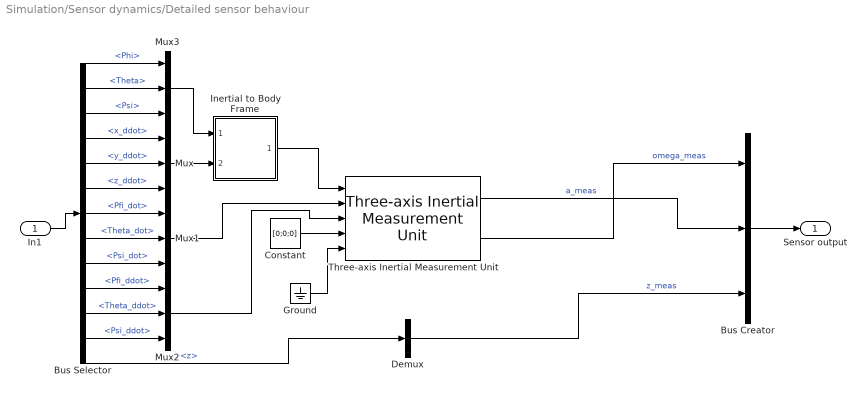
== system Simulation/Sensor dynamics/Detailed sensor behaviour ==
  In1 : Inport
  Bus Creator : BusCreator  Inputs=3
  Bus Selector : BusSelector  OutputSignals=Phi,Theta,Psi,x_ddot,y_ddot,z_ddot,Pfi_dot,Theta_dot,Psi_dot,Pfi_ddot,Theta_ddot,Psi_ddot,z
  Constant : Constant  Value=[0;0;0]
  Demux : Demux  Outputs=1
  Ground : Ground
  Inertial to Body Frame : Subsystem
  Mux{,1..3} (4 alike) : Mux  Inputs=3
  Three-axis Inertial Measurement Unit : aerolibnav/Three-axis Inertial Measurement Unit  units=Metric (MKS)  imu=[0 0 0]  i_Ts=gyro_update_rate  dtype_a=on  w_a=190  z_a=0.707  a_sf_cc=[1 0 0; 0 1 0; 0 0 1]  a_bias=[0 0 0]  a_sat="[-inf  -inf  -inf  inf inf inf]"  dtype_g=on  w_g=190  z_g=0.707  g_sf_cc=[1 0 0; 0 1 0; 0 0 1]  g_bias=[0 0 0]  g_sens=[0 0 0]  g_sat="[-inf  -inf  -inf  inf inf inf]"  i_rand=on  i_seeds=[23093 23094 23095 23096 23097 23098]  i_pow=[0.001 0.001 0.001 0.0001 0.0001 0.0001]
  Sensor output : Outport
  wires:
  Constant/1 -> Three-axis Inertial Measurement Unit/4
  Bus Selector/8 -> Mux1/2  "<Theta_dot>"
  Bus Selector/10 -> Mux2/1  "<Pfi_ddot>"
  Bus Selector/7 -> Mux1/1  "<Pfi_dot>"
  Bus Selector/5 -> Mux/2  "<y_ddot>"
  Bus Selector/12 -> Mux2/3  "<Psi_ddot>"
  Bus Selector/11 -> Mux2/2  "<Theta_ddot>"
  Bus Creator/1 -> Sensor output/1
  Three-axis Inertial Measurement Unit/1 -> Bus Creator/2  "a_meas"
  Three-axis Inertial Measurement Unit/2 -> Bus Creator/1  "omega_meas"
  Bus Selector/13 -> Demux/1  "<z>"
  Bus Selector/9 -> Mux1/3  "<Psi_dot>"
  Bus Selector/4 -> Mux/1  "<x_ddot>"
  Mux1/1 -> Three-axis Inertial Measurement Unit/2
  Mux2/1 -> Three-axis Inertial Measurement Unit/3
  Demux/1 -> Bus Creator/3  "z_meas"
  In1/1 -> Bus Selector/1
  Ground/1 -> Three-axis Inertial Measurement Unit/5
  Bus Selector/6 -> Mux/3  "<z_ddot>"
  Inertial to Body Frame/1(Body Vector) -> Three-axis Inertial Measurement Unit/1
  Bus Selector/1 -> Mux3/1  "<Phi>"
  Bus Selector/2 -> Mux3/2  "<Theta>"
  Bus Selector/3 -> Mux3/3  "<Psi>"
  Mux3/1 -> Inertial to Body Frame/1(Angles)
  Mux/1 -> Inertial to Body Frame/2(Inertial Vector)

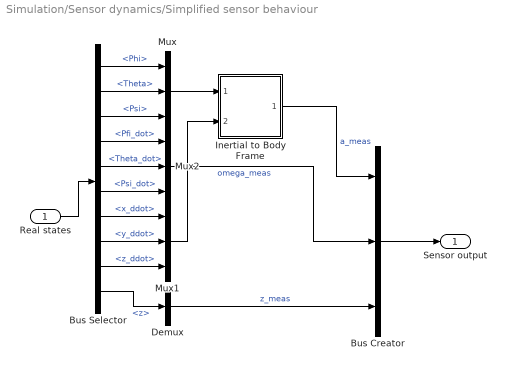
== system Simulation/Sensor dynamics/Simplified sensor behaviour ==
  Real states : Inport
  Bus Creator : BusCreator  Inputs=3
  Bus Selector : BusSelector  OutputSignals=Phi,Theta,Psi,Pfi_dot,Theta_dot,Psi_dot,x_ddot,y_ddot,z_ddot,z
  Demux : Demux  Outputs=1
  Inertial to Body Frame : Subsystem
  Mux : Mux  Inputs=3
  Mux1 : Mux  Inputs=3
  Mux2 : Mux  Inputs=3
  Sensor output : Outport
  wires:
  Bus Selector/5 -> Mux2/2  "<Theta_dot>"
  Bus Selector/10 -> Demux/1  "<z>"
  Bus Selector/7 -> Mux1/1  "<x_ddot>"
  Bus Selector/9 -> Mux1/3  "<z_ddot>"
  Bus Selector/4 -> Mux2/1  "<Pfi_dot>"
  Bus Selector/6 -> Mux2/3  "<Psi_dot>"
  Bus Creator/1 -> Sensor output/1
  Real states/1 -> Bus Selector/1
  Bus Selector/8 -> Mux1/2  "<y_ddot>"
  Demux/1 -> Bus Creator/3  "z_meas"
  Bus Selector/3 -> Mux/3  "<Psi>"
  Bus Selector/1 -> Mux/1  "<Phi>"
  Bus Selector/2 -> Mux/2  "<Theta>"
  Mux/1 -> Inertial to Body Frame/1(Angles)
  Mux1/1 -> Inertial to Body Frame/2(Inertial Vector)
  Inertial to Body Frame/1(Body Vector) -> Bus Creator/1  "a_meas"
  Mux2/1 -> Bus Creator/2  "omega_meas"

== system Simulation/State estimator/Ideal State estimator ==
  In1 : Inport
  Bus Creator2 : BusCreator  Inputs=6
  Bus Selector : BusSelector  OutputSignals=a_meas,z_meas,omega_meas
  Demux : Demux  Outputs=3
  Demux1 : Demux  Outputs=3
  Demux2 : Demux  Outputs=1
  Integrator : Integrator
  Integrator1 : Integrator
  Out1 : Outport
  wires:
  In1/1 -> Bus Selector/1
  Bus Creator2/1 -> Out1/1
  Bus Selector/1 -> Integrator/1  "<a_meas>"
  Integrator/1 -> Demux/1
  Demux/1 -> Bus Creator2/1  "x_est"
  Demux/2 -> Bus Creator2/2  "y_est"
  Bus Selector/3 -> Integrator1/1  "<omega_meas>"
  Integrator1/1 -> Demux1/1
  Demux1/1 -> Bus Creator2/4  "Pfi_est"
  Demux1/2 -> Bus Creator2/5  "Theta_est"
  Demux1/3 -> Bus Creator2/6  "Psi_est"
  Demux2/1 -> Bus Creator2/3  "z_est"
  Bus Selector/2 -> Demux2/1  "<z_meas>"

== system Simulation/Controller/Attitude and z control/Other method ==
  Desired States : Inport
  Estimated States : Inport  Port=2
  Action Port : ActionPort  ActionPortLabel=else
  Constant : Constant
  Mux : Mux
  Out1 : Outport
  wires:
  Constant/1 -> Mux/2, Mux/1, Mux/4, Mux/3
  Mux/1 -> Out1/1

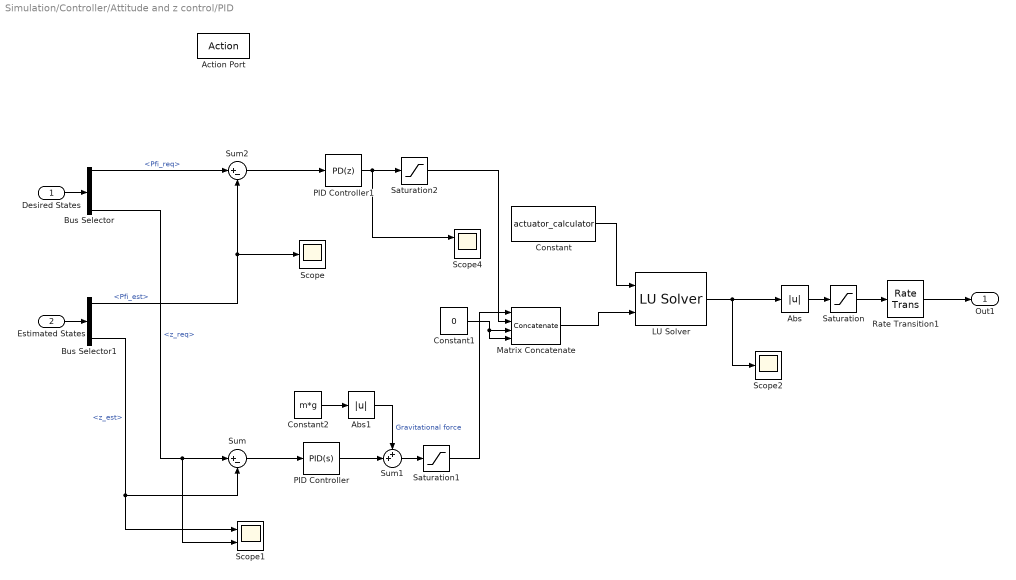
== system Simulation/Controller/Attitude and z control/PID ==
  Desired States : Inport
  Estimated States : Inport  Port=2
  Action Port : ActionPort  ActionPortLabel=if(u1 == 0)
  Abs : Abs
  Abs1 : Abs
  Bus Selector : BusSelector  OutputSignals=Pfi_req,Theta_req,Psi_req,z_req
  Bus Selector1 : BusSelector  OutputSignals=Pfi_est,y_est,z_est
  Constant : Constant  Value=actuator_calculator
  Constant1 : Constant  Value=0
  Constant2 : Constant  Value=m*g
  LU Solver : dspsolvers/LU Solver
      settings: SourceProductName=DSP System Toolbox  SourceProductBaseCode=DS
  Matrix Concatenate : Concatenate  NumInputs=4
  PID Controller : simulink/Continuous/PID Controller  Controller=PID  Form=Parallel  TimeDomain=Continuous-time  SampleTime=-1  IntegratorMethod=Forward Euler  FilterMethod=Forward Euler  ControllerParametersSource=internal  P=0.22  I=0.000000001  D=0.65  UseFilter=on  N=100  TunerSelectOption=Transfer Function Based (PID Tuner App)  InitialConditionSource=internal  InitialConditionForIntegrator=0  InitialConditionForFilter=0  DifferentiatorICPrevScaledInput=0  ExternalReset=none  TrackingMode=off  Kt=1  LimitOutput=off  UpperSaturationLimit=inf  LowerSaturationLimit=-inf  LinearizeAsGain=on  AntiWindupMode=none  Kb=1  POutMin=[]  POutMax=[]  IOutMin=[]  IOutMax=[]  DOutMin=[]  DOutMax=[]  NOutMin=[]  NOutMax=[]  SumOutMin=[]  SumOutMax=[]  SaturationOutMin=[]  SaturationOutMax=[]  PParamMin=[]  PParamMax=[]  IParamMin=[]  IParamMax=[]  DParamMin=[]  DParamMax=[]  NParamMin=[]  NParamMax=[]  KbParamMin=[]  KbParamMax=[]  KtParamMin=[]  KtParamMax=[]  KbOutMin=[]  KbOutMax=[]  KtOutMin=[]  KtOutMax=[]  IntegratorOutMin=[]  IntegratorOutMax=[]  FilterOutMin=[]  FilterOutMax=[]  SumI1OutMin=[]  SumI1OutMax=[]  SumI2OutMin=[]  SumI2OutMax=[]  SumI3OutMin=[]  SumI3OutMax=[]  SumI4OutMin=[]  SumI4OutMax=[]  SumDOutMin=[]  SumDOutMax=[]  DifferentiatorOutMin=[]  DifferentiatorOutMax=[]  FilterDiffOutCoefMin=[]  FilterDiffOutCoefMax=[]  ReciprocalOutMin=[]  ReciprocalOutMax=[]  SumDenOutMin=[]  SumDenOutMax=[]  SumNumOutMin=[]  SumNumOutMax=[]  DivideOutMin=[]  DivideOutMax=[]  IntegratorContinuousStateAttributes=''  IntegratorStateMustResolveToSignalObject=off  IntegratorRTWStateStorageClass=Auto  FilterContinuousStateAttributes=''  FilterStateMustResolveToSignalObject=off  FilterRTWStateStorageClass=Auto  ParallelPVariant=InternalParameters  IdealPVariant=Disabled  IVariant=InternalParameters  DVariant=InternalParameters  IntegratorVariant=Continuous  SatVariant=Disabled  AWVariant=Passthrough  PCopyVariant=Disabled  TRVariant=Disabled  FdbkBlocksVariant=Forward  IdealPFdbkVariant=Disabled  SatFdbkVariant=Disabled  DerivativeFilterVariant=ContFilter  NVariant=InternalParameters  NCopyVariant=Disabled  FilterICVariant=InternalICsFilter  IntegratorICVariant=InternalICs  ExternalResetVariant=Disabled  TRSumVariant=Passthrough  SumFdbkVariant=Disabled  SumVariant=Sum_PID
  PID Controller1 : simulink/Continuous/PID Controller  Controller=PD  Form=Parallel  TimeDomain=Discrete-time  SampleTime=0.01  IntegratorMethod=Forward Euler  FilterMethod=Forward Euler  ControllerParametersSource=internal  P=0.00259411107130878  I=0  D=0  UseFilter=on  N=36.9920183842659  TunerSelectOption=Transfer Function Based (PID Tuner App)  InitialConditionSource=internal  InitialConditionForIntegrator=0  InitialConditionForFilter=0  DifferentiatorICPrevScaledInput=0  ExternalReset=none  TrackingMode=off  Kt=1  LimitOutput=off  UpperSaturationLimit=inf  LowerSaturationLimit=-inf  LinearizeAsGain=on  AntiWindupMode=none  Kb=1  POutMin=[]  POutMax=[]  IOutMin=[]  IOutMax=[]  DOutMin=[]  DOutMax=[]  NOutMin=[]  NOutMax=[]  SumOutMin=[]  SumOutMax=[]  SaturationOutMin=[]  SaturationOutMax=[]  PParamMin=[]  PParamMax=[]  IParamMin=[]  IParamMax=[]  DParamMin=[]  DParamMax=[]  NParamMin=[]  NParamMax=[]  KbParamMin=[]  KbParamMax=[]  KtParamMin=[]  KtParamMax=[]  KbOutMin=[]  KbOutMax=[]  KtOutMin=[]  KtOutMax=[]  IntegratorOutMin=[]  IntegratorOutMax=[]  FilterOutMin=[]  FilterOutMax=[]  SumI1OutMin=[]  SumI1OutMax=[]  SumI2OutMin=[]  SumI2OutMax=[]  SumI3OutMin=[]  SumI3OutMax=[]  SumI4OutMin=[]  SumI4OutMax=[]  SumDOutMin=[]  SumDOutMax=[]  DifferentiatorOutMin=[]  DifferentiatorOutMax=[]  FilterDiffOutCoefMin=[]  FilterDiffOutCoefMax=[]  ReciprocalOutMin=[]  ReciprocalOutMax=[]  SumDenOutMin=[]  SumDenOutMax=[]  SumNumOutMin=[]  SumNumOutMax=[]  DivideOutMin=[]  DivideOutMax=[]  IntegratorContinuousStateAttributes=''  IntegratorStateMustResolveToSignalObject=off  IntegratorRTWStateStorageClass=Auto  FilterContinuousStateAttributes=''  FilterStateMustResolveToSignalObject=off  FilterRTWStateStorageClass=Auto  ParallelPVariant=InternalParameters  IdealPVariant=Disabled  IVariant=Disabled  DVariant=InternalParameters  IntegratorVariant=Disabled  SatVariant=Disabled  AWVariant=Disabled  PCopyVariant=Disabled  TRVariant=Disabled  FdbkBlocksVariant=Forward  IdealPFdbkVariant=Disabled  SatFdbkVariant=Disabled  DerivativeFilterVariant=ForwardEulerFilter  NVariant=InternalParameters  NCopyVariant=Disabled  FilterICVariant=InternalICsFilter  IntegratorICVariant=Disabled  ExternalResetVariant=Disabled  TRSumVariant=Passthrough  SumFdbkVariant=Disabled  SumVariant=Sum_PD
  Rate Transition1 : RateTransition
  Saturation : Saturate  UpperLimit=maxLiftForce  LowerLimit=0
  Saturation1 : Saturate  UpperLimit=4 * maxLiftForce  LowerLimit=0
  Saturation2 : Saturate
  Scope : Scope
  Scope1 : Scope  NumInputPorts=2
  Scope2 : Scope
  Scope4 : Scope  NumInputPorts=2
  Sum : Sum  Inputs=|+-
  Sum1 : Sum  Inputs=++|
  Sum2 : Sum  Inputs=|+-
  Out1 : Outport
  wires:
  Desired States/1 -> Bus Selector/1
  Estimated States/1 -> Bus Selector1/1
  LU Solver/1 -> Scope2/1, Abs/1
  Abs/1 -> Saturation/1
  Constant/1 -> LU Solver/1
  Matrix Concatenate/1 -> LU Solver/2
  Sum/1 -> PID Controller/1
  Bus Selector/4 -> Scope1/2, Sum/1  "<z_req>"
  Bus Selector1/3 -> Scope1/1, Sum/2  "<z_est>"
  Constant1/1 -> Matrix Concatenate/3, Matrix Concatenate/4
  Sum1/1 -> Saturation1/1
  Constant2/1 -> Abs1/1
  Abs1/1 -> Sum1/1  "Gravitational force"
  PID Controller/1 -> Sum1/2
  Saturation1/1 -> Matrix Concatenate/1
  Saturation/1 -> Rate Transition1/1
  Bus Selector/1 -> Sum2/1  "<Pfi_req>"
  Bus Selector1/1 -> Scope/1, Sum2/2  "<Pfi_est>"
  Sum2/1 -> PID Controller1/1
  PID Controller1/1 -> Scope4/1, Saturation2/1
  Saturation2/1 -> Matrix Concatenate/2
  Rate Transition1/1 -> Out1/1

== system Simulation/Controller/PID Attitude-Altitude controller/Inertial to Body Frame ==
  Angles : Inport
  Inertial Vector : Inport  Port=2
  Matrix Multiply : Product  Multiplication=Matrix(*)
  Rotation Angles to Direction Cosine Matrix : sharedtransform/Rotation Angles to Direction Cosine Matrix  rotationOrder=ZYX  aMode=aMode
      settings: SourceProductBaseCode=AE
  Selector3 : Selector  InputPortWidth=3  IndexOptions=Index vector (dialog)  Indices=[3 2 1]  OutputSizes=1
  Body Vector : Outport
  wires:
  Selector3/1 -> Rotation Angles to Direction Cosine Matrix/1
  Angles/1 -> Selector3/1
  Matrix Multiply/1 -> Body Vector/1
  Inertial Vector/1 -> Matrix Multiply/2
  Rotation Angles to Direction Cosine Matrix/1 -> Matrix Multiply/1

== system Simulation/Controller/Position Control/Method 2 ==
  Desired State : Inport
  Estimated State : Inport  Port=2
  Action Port : ActionPort  ActionPortLabel=else
  Constant : Constant
  Mux : Mux
  Output : Outport
  wires:
  Mux/1 -> Output/1
  Constant/1 -> Mux/2, Mux/1, Mux/4, Mux/3

== system Simulation/Controller/Position Control/PID ==
  Desired State : Inport
  Estimated State : Inport  Port=2
  Action Port : ActionPort  ActionPortLabel=if(u1 == 0)
  Bus Selector : BusSelector  OutputSignals=x_req,y_req,z_req
  Bus Selector1 : BusSelector  OutputSignals=x_est,y_est,z_est
  Constant : Constant
  Mux : Mux
  Output : Outport
  wires:
  Desired State/1 -> Bus Selector/1
  Estimated State/1 -> Bus Selector1/1
  Constant/1 -> Mux/2, Mux/1, Mux/4, Mux/3
  Mux/1 -> Output/1

== system Simulation/Sensor dynamics/Detailed sensor behaviour/Inertial to Body Frame ==
  Angles : Inport
  Inertial Vector : Inport  Port=2
  Matrix Multiply : Product  Multiplication=Matrix(*)
  Rotation Angles to Direction Cosine Matrix : sharedtransform/Rotation Angles to Direction Cosine Matrix  rotationOrder=ZYX  aMode=aMode
      settings: SourceProductBaseCode=AE
  Selector3 : Selector  InputPortWidth=3  IndexOptions=Index vector (dialog)  Indices=[3 2 1]  OutputSizes=1
  Body Vector : Outport
  wires:
  Selector3/1 -> Rotation Angles to Direction Cosine Matrix/1
  Angles/1 -> Selector3/1
  Matrix Multiply/1 -> Body Vector/1
  Inertial Vector/1 -> Matrix Multiply/2
  Rotation Angles to Direction Cosine Matrix/1 -> Matrix Multiply/1

== system Simulation/Sensor dynamics/Simplified sensor behaviour/Inertial to Body Frame ==
  Angles : Inport
  Inertial Vector : Inport  Port=2
  Matrix Multiply : Product  Multiplication=Matrix(*)
  Rotation Angles to Direction Cosine Matrix : sharedtransform/Rotation Angles to Direction Cosine Matrix  rotationOrder=ZYX  aMode=aMode
      settings: SourceProductBaseCode=AE
  Selector3 : Selector  InputPortWidth=3  IndexOptions=Index vector (dialog)  Indices=[3 2 1]  OutputSizes=1
  Body Vector : Outport
  wires:
  Selector3/1 -> Rotation Angles to Direction Cosine Matrix/1
  Angles/1 -> Selector3/1
  Matrix Multiply/1 -> Body Vector/1
  Inertial Vector/1 -> Matrix Multiply/2
  Rotation Angles to Direction Cosine Matrix/1 -> Matrix Multiply/1
